simulink model "linear_model"  (R2020b)
settings: Solver=FixedStepAuto  StartTime=0.0  StopTime=5  FixedStep=0.0001  RelTol=1e-3
values from neighbouring files (symbols this model uses):
  B = 3.4    [nonlinear_quicktest.m]
  cont_den = cont_den_master    [nonlinear_quicktest.m]
  cont_num = cont_num_master    [nonlinear_quicktest.m]
  J_eq = J_1 + n_1^2 *(J_2 + M_3*r_3^2)    (= 2.88733377778e-05)    [nonlinear_quicktest.m]
  K_tau = 42e-3    (= 0.042)    [nonlinear_quicktest.m]
  n_1 = 1/3    (= 0.333333333333)    [nonlinear_quicktest.m]
  r_3 = 0.0127    [nonlinear_quicktest.m]
  step_size = step_size_array(j)    [main.m]    (also in nonlinear_quicktest.m = 0.1; span_optimering_quicker.m = 1)
settings Model: Creator=Bens PC  LastModifiedBy=Bens PC

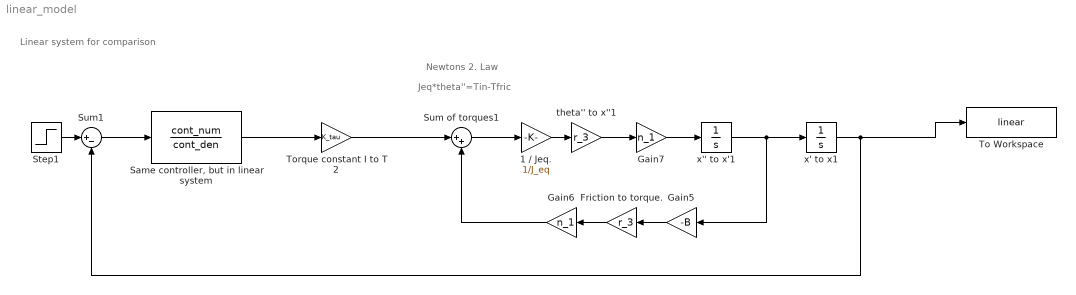
== system linear_model ==
  note: Linear system for comparison
  note: Jeq*theta''=Tin-Tfric
  note: Newtons 2. Law
  1 / Jeq. : Gain  Gain=1/J_eq
  Friction to torque. : Gain  Gain=r_3
  Gain5 : Gain  Gain=-B
  Gain6 : Gain  Gain=n_1
  Gain7 : Gain  Gain=n_1
  "Same controller, but in linear system" : TransferFcn  Numerator=cont_num  Denominator=cont_den
  Step1 : Step  Time=0  After=step_size  SampleTime=0
  Sum of torques1 : Sum  Inputs=|++
  Sum1 : Sum  Inputs=|+-
  To Workspace : ToWorkspace  VariableName=linear  SaveFormat=Timeseries  SampleTime=-1
  Torque constant I to T 2 : Gain  Gain=K_tau
  theta'' to x''1 : Gain  Gain=r_3
  x' to x1 : Integrator
  x'' to x'1 : Integrator
  wires:
  "Same controller, but in linear system"/1 -> Torque constant I to T 2/1
  Torque constant I to T 2/1 -> Sum of torques1/1
  Sum of torques1/1 -> 1 / Jeq./1
  1 / Jeq./1 -> theta'' to x''1/1
  x' to x1/1 -> To Workspace/1, Sum1/2
  x'' to x'1/1 -> Gain5/1, x' to x1/1
  Gain5/1 -> Friction to torque./1
  Sum1/1 -> "Same controller, but in linear system"/1
  Gain6/1 -> Sum of torques1/2
  Friction to torque./1 -> Gain6/1
  Step1/1 -> Sum1/1
  theta'' to x''1/1 -> Gain7/1
  Gain7/1 -> x'' to x'1/1
